simulink model "W07_Design_Verify"  (R2024b)
settings: Solver=ode45  StartTime=0.0  StopTime=t_end2  MaxStep=0.01  RelTol=1e-3
PreLoadFcn:
  | % W07_Design_Verify 기본 파라미터 (모델을 열 때 자동 실행)
  | % 플랜트 G(s) = 1 / (s(s+2)(s+5))
  | defs = { 'K_des',4.79 ; 'u_lim',5 ; 't_end2',12 ;
  |          'numG2',1 ; 'denG2',[1 7 10 0] };
  | for ii = 1:size(defs,1)
  |     if ~evalin('base', sprintf('exist(''%s'',''var'')', defs{ii,1}))
  |         assignin('base', defs{ii,1}, defs{ii,2});
  |     end
  | end
  | clear defs ii
values from neighbouring files (symbols this model uses):
  denG2 = [1 7 10 0]    [W07_06_run_simulink.m]
  K_des = 4.79    [W07_06_run_simulink.m]
  numG2 = 1    [W07_06_run_simulink.m]
  u_lim = 5    [W07_06_run_simulink.m]
settings Model: Creator=admin  LastModifiedBy=admin

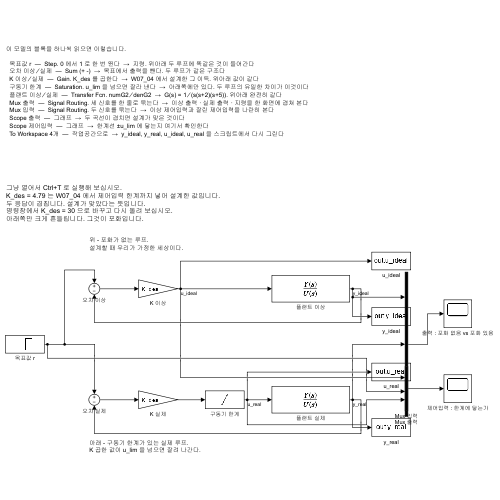
[thumbnail: Simulink's stored preview of the top-level diagram]
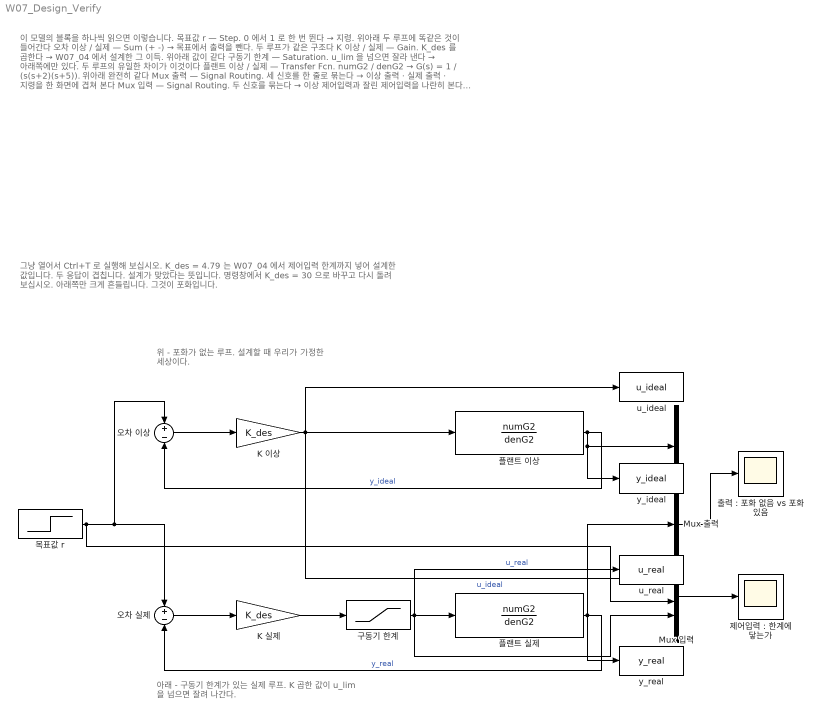
== system W07_Design_Verify ==
  note: 위 - 포화가 없는 루프.
      | 설계할 때 우리가 가정한 세상이다.
  note: 아래 - 구동기 한계가 있는 실제 루프.
      | K 곱한 값이 u_lim 을 넘으면 잘려 나간다.
  note: 그냥 열어서 Ctrl+T 로 실행해 보십시오.
      | K_des = 4.79 는 W07_04 에서 제어입력 한계까지 넣어 설계한 값입니다.
      | 두 응답이 겹칩니다. 설계가 맞았다는 뜻입니다.
      | 명령창에서 K_des = 30 으로 바꾸고 다시 돌려 보십시오.
      | 아래쪽만 크게 흔들립니다. 그것이 포화입니다.
  note: 이 모델의 블록을 하나씩 읽으면 이렇습니다.
      |
      |   목표값 r  —  Step. 0 에서 1 로 한 번 뛴다  →  지령. 위아래 두 루프에 똑같은 것이 들어간다
      |   오차 이상 ∕ 실제  —  Sum (+ -)  →  목표에서 출력을 뺀다. 두 루프가 같은 구조다
      |   K 이상 ∕ 실제  —  Gain. K_des 를 곱한다  →  W07_04 에서 설계한 그 이득. 위아래 값이 같다
      |   구동기 한계  —  Saturation. u_lim 을 넘으면 잘라 낸다  →  아래쪽에만 있다. 두 루프의 유일한 차이가 이것이다
      |   플랜트 이상 ∕ 실제  —  Transfer Fcn. numG2 ∕ denG2  →  G(s) = 1 ∕ (s(s+2)(s+5)). 위아래 완전히 같다
      |   Mux 출력  —  Signal Routing. 세 신호를 한 줄로 묶는다  →  이상 출력 · 실제 출력 · 지령을 한 화면에 겹쳐 본다
      |   Mux 입력  —  Signal Routing. 두 신호를 묶는다  →  이상 제어입력과 잘린 제어입력을 나란히 본다
      |   Scope 출력  —  그래프  →  두 곡선이 겹치면 설계가 맞은 것이다
      |   Scope 제어입력  —  그래프  →  한계선 ±u_lim 에 닿는지 여기서 확인한다
      |   To Workspace 4개  —  작업공간으로  →  y_ideal, y_real, u_ideal, u_real 을 스크립트에서 다시 그린다
  K 실제 : Gain  Gain=K_des
  K 이상 : Gain  Gain=K_des
  Mux 입력 : Mux  Inputs=2
  Mux 출력 : Mux  Inputs=3
  u_ideal : ToWorkspace  VariableName=u_ideal  SaveFormat=Timeseries  SampleTime=-1
  u_real : ToWorkspace  VariableName=u_real  SaveFormat=Timeseries  SampleTime=-1
  y_ideal : ToWorkspace  VariableName=y_ideal  SaveFormat=Timeseries  SampleTime=-1
  y_real : ToWorkspace  VariableName=y_real  SaveFormat=Timeseries  SampleTime=-1
  구동기 한계 : Saturate  UpperLimit=u_lim  LowerLimit=-u_lim
  목표값 r : Step  Time=0  SampleTime=0
  오차 실제 : Sum  Inputs=+-
  오차 이상 : Sum  Inputs=+-
  "제어입력 : 한계에 닿는가" : Scope
  "출력 : 포화 없음 vs 포화 있음" : Scope
  플랜트 실제 : TransferFcn  Numerator=numG2  Denominator=denG2
  플랜트 이상 : TransferFcn  Numerator=numG2  Denominator=denG2
  wires:
  목표값 r/1 -> 오차 이상/1, 오차 실제/1, Mux 출력/3
  오차 이상/1 -> K 이상/1
  K 이상/1 -> 플랜트 이상/1, u_ideal/1, Mux 입력/1  "u_ideal"
  플랜트 이상/1 -> y_ideal/1, Mux 출력/1, 오차 이상/2  "y_ideal"
  오차 실제/1 -> K 실제/1
  K 실제/1 -> 구동기 한계/1
  구동기 한계/1 -> 플랜트 실제/1, u_real/1, Mux 입력/2  "u_real"
  플랜트 실제/1 -> 오차 실제/2, y_real/1, Mux 출력/2  "y_real"
  Mux 출력/1 -> "출력 : 포화 없음 vs 포화 있음"/1
  Mux 입력/1 -> "제어입력 : 한계에 닿는가"/1
